simulink model "control_simulator"  (R2024b)
settings: Solver=FixedStepDiscrete  StartTime=0.0  StopTime=45  FixedStep=0.01  RelTol=1e-3
values from neighbouring files (symbols this model uses):
  Kd_dote = 0    [controller_params.m]
  Kd_dotp = 0    [controller_params.m]
  Kd_dott = 0.2    [controller_params.m]
  Kd_e = 0    [controller_params.m]
  Kd_p = 1    [controller_params.m]
  Kd_t = 0.16    [controller_params.m]
  Ki_dote = 10    [controller_params.m]
  Ki_dotp = 1.2    [controller_params.m]
  Ki_dott = 0.05    [controller_params.m]
  Ki_e = 0    [controller_params.m]
  Ki_p = 0    [controller_params.m]
  Ki_t = 0.0    (= 0)    [controller_params.m]
  Kp_dote = 5    [controller_params.m]
  Kp_dotp = 3.8    [controller_params.m]
  Kp_dott = 0.3    [controller_params.m]
  Kp_e = 1.5    [controller_params.m]
  Kp_p = 1.5    [controller_params.m]
  Kp_t = 0.4    [controller_params.m]
  max_dote = 4    [controller_params.m]
  max_dotp = 3    [controller_params.m]
  max_dott = deg2rad(15)    [controller_params.m]
  max_e = deg2rad(45)    [controller_params.m]
  max_p = deg2rad(45)    [controller_params.m]
  max_t = deg2rad(45)    [controller_params.m]
  min_dote = 0    [controller_params.m]
  min_dotp = -3    [controller_params.m]
  min_dott = -deg2rad(15)    [controller_params.m]
  min_e = -deg2rad(45)    [controller_params.m]
  min_p = -deg2rad(45)    [controller_params.m]
  min_t = -deg2rad(45)    [controller_params.m]
libraries: slpidlib x6
settings Model: Creator=bryankikuta  LastModifiedBy=bryankikuta

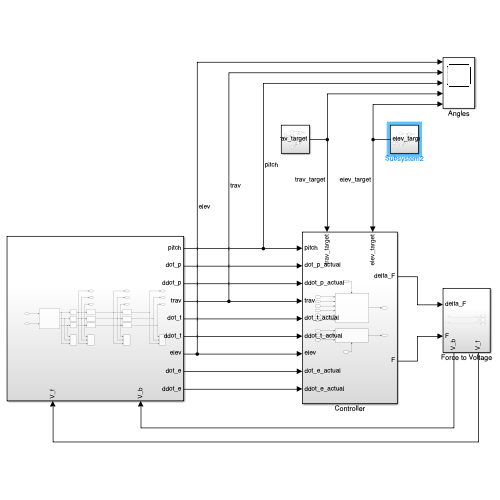
[thumbnail: Simulink's stored preview of the top-level diagram]
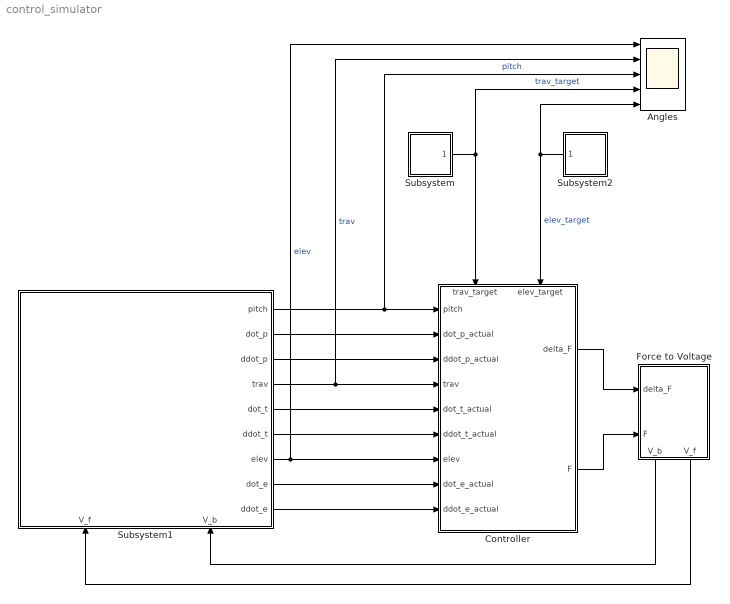
== system control_simulator ==
  Angles : Scope  NumInputPorts=5
  Controller : Subsystem
      settings: PortSchema="{\"entries\":[{\"content\":{\"sides\":[{\"content\":{\"connectorIds\":[\"In1\",\"In2\",\"In3\",\"In4\",\"In5\",\"In6\",\"In7\",\"In8\",\"In9\"]},\"type\":\"ConnectorPlacement.EquallySpacedRectSide\",\"uuid\":\"b9be8901-0178-4093-bc1f-7a19329e3ddd\"},{\"content\":{\"connectorIds\":[\"Out1\",\"Out2\"],\"side\":\"RIGHT\"},\"type\":\"ConnectorPlacement.EquallySpacedRectSide\",\"uuid\":\"79e1f72b-8678-4c9d-874f-f1aeb3aff2e8\"},{\"content\":{\"connectorIds\":[\"In10\",\"In11\"],\"side\":\"TOP\"},\"type\":\"ConnectorPlacement.EquallySpacedRectSide\",\"uuid\":\"c11cbc2b-c46d-45de-b9fa-5f1631f2c60a\"}]},\"type\":\"ConnectorPlacement.EquallySpacedConnector\",\"uuid\":\"5eabee5a-01a3-4056-9340-8a43b1588280\"}],\"packageUris\":[\"http://schema.mathworks.com/mf0/Connector/R2020b\"],\"version\":\"1.0\"}"
  Force to Voltage : Subsystem
      settings: PortSchema="{\"entries\":[{\"content\":{\"sides\":[{\"content\":{\"connectorIds\":[\"In1\",\"In2\"]},\"type\":\"ConnectorPlacement.EquallySpacedRectSide\",\"uuid\":\"6f137349-bbac-4947-af72-a88291b00c32\"},{\"content\":{\"side\":\"RIGHT\"},\"type\":\"ConnectorPlacement.EquallySpacedRectSide\",\"uuid\":\"62cbe85c-e78c-4219-9070-536950e9188e\"},{\"content\":{\"side\":\"TOP\"},\"type\":\"ConnectorPlacement.EquallySpacedRectSide\",\"uuid\":\"b2b4bc51-a272-402c-9560-9dda5e41a8e7\"},{\"content\":{\"connectorIds\":[\"Out1\",\"Out2\"],\"side\":\"BOTTOM\"},\"type\":\"ConnectorPlacement.EquallySpacedRectSide\",\"uuid\":\"97d29757-9418-4318-9369-020d2350e0e0\"}]},\"type\":\"ConnectorPlacement.EquallySpacedConnector\",\"uuid\":\"58f565a6-402e-4fc1-b947-4e751bcba226\"}],\"packageUris\":[\"http://schema.mathworks.com/mf0/Connector/R2020b\"],\"version\":\"1.0\"}"
  Subsystem : Subsystem
  Subsystem1 : Subsystem
      settings: PortSchema="{\"entries\":[{\"content\":{\"sides\":[{\"content\":{},\"type\":\"ConnectorPlacement.EquallySpacedRectSide\",\"uuid\":\"85796e1e-dc7e-47a4-94ca-9dbd2389fb42\"},{\"content\":{\"connectorIds\":[\"Out1\",\"Out2\",\"Out3\",\"Out4\",\"Out5\",\"Out6\",\"Out7\",\"Out8\",\"Out9\"],\"side\":\"RIGHT\"},\"type\":\"ConnectorPlacement.EquallySpacedRectSide\",\"uuid\":\"0966b95d-a260-4754-9670-31181c58c2b3\"},{\"content\":{\"side\":\"TOP\"},\"type\":\"ConnectorPlacement.EquallySpacedRectSide\",\"uuid\":\"e674cd1b-7e3a-4241-b627-b9ea271cb489\"},{\"content\":{\"connectorIds\":[\"In1\",\"In2\"],\"side\":\"BOTTOM\"},\"type\":\"ConnectorPlacement.EquallySpacedRectSide\",\"uuid\":\"4a7c60fe-460d-4522-942d-cbc66a60857c\"}]},\"type\":\"ConnectorPlacement.EquallySpacedConnector\",\"uuid\":\"488257c1-7be2-46d6-bbfb-c75cce3631e5\"}],\"packageUris\":[\"http://schema.mathworks.com/mf0/Connector/R2020b\"],\"version\":\"1.0\"}"
  Subsystem2 : Subsystem
      settings: PortSchema="{\"entries\":[{\"content\":{\"sides\":[{\"content\":{\"connectorIds\":[\"Out1\"]},\"type\":\"ConnectorPlacement.EquallySpacedRectSide\",\"uuid\":\"f16ebcfb-7c7e-48d0-898d-d7ef16663e42\"},{\"content\":{\"side\":\"RIGHT\"},\"type\":\"ConnectorPlacement.EquallySpacedRectSide\",\"uuid\":\"e9aec1bf-af4d-4e60-94a2-adac9fbe53b1\"},{\"content\":{\"side\":\"TOP\"},\"type\":\"ConnectorPlacement.EquallySpacedRectSide\",\"uuid\":\"bae62bc1-b0f5-4305-8efd-ec446c0d0572\"}]},\"type\":\"ConnectorPlacement.EquallySpacedConnector\",\"uuid\":\"f37ab34b-dfa4-4a7d-8642-621e1edbbf7a\"}],\"packageUris\":[\"http://schema.mathworks.com/mf0/Connector/R2020b\"],\"version\":\"1.0\"}"
  wires:
  Subsystem1/1(pitch) -> Angles/3, Controller/1(pitch)  "pitch"
  Subsystem1/4(trav) -> Angles/2, Controller/4(trav)  "trav"
  Subsystem1/7(elev) -> Angles/1, Controller/7(elev)  "elev"
  Force to Voltage/2(V_f) -> Subsystem1/1(V_f)
  Force to Voltage/1(V_b) -> Subsystem1/2(V_b)
  Subsystem1/2(dot_p) -> Controller/2(dot_p_actual)
  Subsystem1/3(ddot_p) -> Controller/3(ddot_p_actual)
  Subsystem1/5(dot_t) -> Controller/5(dot_t_actual)
  Subsystem1/6(ddot_t) -> Controller/6(ddot_t_actual)
  Subsystem1/8(dot_e) -> Controller/8(dot_e_actual)
  Subsystem1/9(ddot_e) -> Controller/9(ddot_e_actual)
  Controller/1(delta_F) -> Force to Voltage/1(delta_F)
  Controller/2(F) -> Force to Voltage/2(F)
  Subsystem/1(trav_target) -> Angles/4, Controller/10(trav_target)  "trav_target"
  Subsystem2/1(elev_target) -> Controller/11(elev_target), Angles/5  "elev_target"

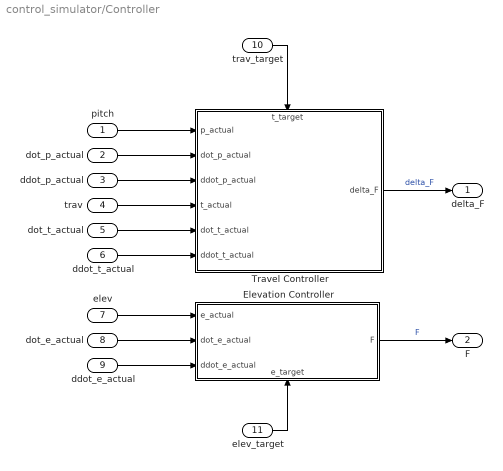
== system control_simulator/Controller ==
  pitch : Inport
  dot_p_actual : Inport  Port=2
  ddot_p_actual : Inport  Port=3
  trav : Inport  Port=4
  dot_t_actual : Inport  Port=5
  ddot_t_actual : Inport  Port=6
  elev : Inport  Port=7
  dot_e_actual : Inport  Port=8
  ddot_e_actual : Inport  Port=9
  trav_target : Inport  Port=10
  elev_target : Inport  Port=11
  Elevation Controller : Subsystem
      settings: PortSchema="{\"entries\":[{\"content\":{\"sides\":[{\"content\":{\"connectorIds\":[\"In1\",\"In2\",\"In3\"]},\"type\":\"ConnectorPlacement.EquallySpacedRectSide\",\"uuid\":\"9da0c654-dd8f-4eac-9c62-49b15265654d\"},{\"content\":{\"connectorIds\":[\"Out1\"],\"side\":\"RIGHT\"},\"type\":\"ConnectorPlacement.EquallySpacedRectSide\",\"uuid\":\"bed5ee04-0f93-4f10-b230-05550981109f\"},{\"content\":{\"side\":\"TOP\"},\"type\":\"ConnectorPlacement.EquallySpacedRectSide\",\"uuid\":\"56ea07fe-d553-41da-8d63-69b8e963b388\"},{\"content\":{\"connectorIds\":[\"In4\"],\"side\":\"BOTTOM\"},\"type\":\"ConnectorPlacement.EquallySpacedRectSide\",\"uuid\":\"e6670811-fda1-486d-a98e-2b76a62b4f3e\"}]},\"type\":\"ConnectorPlacement.EquallySpacedConnector\",\"uuid\":\"b3b4161d-49db-4a00-a039-f772733d1a23\"}],\"packageUris\":[\"http://schema.mathworks.com/mf0/Connector/R2020b\"],\"version\":\"1.0\"}"
  Travel Controller : Subsystem
      settings: PortSchema="{\"entries\":[{\"content\":{\"sides\":[{\"content\":{\"connectorIds\":[\"In1\",\"In2\",\"In3\",\"In4\",\"In5\",\"In6\"]},\"type\":\"ConnectorPlacement.EquallySpacedRectSide\",\"uuid\":\"73e9ec17-e7a6-4f85-a13a-6f8910987c35\"},{\"content\":{\"connectorIds\":[\"Out1\"],\"side\":\"RIGHT\"},\"type\":\"ConnectorPlacement.EquallySpacedRectSide\",\"uuid\":\"c5195cd8-79c4-4218-a9bb-56ca77b55f6e\"},{\"content\":{\"connectorIds\":[\"In7\"],\"side\":\"TOP\"},\"type\":\"ConnectorPlacement.EquallySpacedRectSide\",\"uuid\":\"2d754233-a1a1-48e7-852a-7aeefa75e1cb\"}]},\"type\":\"ConnectorPlacement.EquallySpacedConnector\",\"uuid\":\"9648f682-433b-4a20-950d-debe9f6c7fac\"}],\"packageUris\":[\"http://schema.mathworks.com/mf0/Connector/R2020b\"],\"version\":\"1.0\"}"
  delta_F : Outport
  F : Outport  Port=2
  wires:
  trav_target/1 -> Travel Controller/7(t_target)
  pitch/1 -> Travel Controller/1(p_actual)
  dot_t_actual/1 -> Travel Controller/5(dot_t_actual)
  ddot_p_actual/1 -> Travel Controller/3(ddot_p_actual)
  elev/1 -> Elevation Controller/1(e_actual)
  dot_p_actual/1 -> Travel Controller/2(dot_p_actual)
  Travel Controller/1(delta_F) -> delta_F/1  "delta_F"
  Elevation Controller/1(F) -> F/1  "F"
  dot_e_actual/1 -> Elevation Controller/2(dot_e_actual)
  trav/1 -> Travel Controller/4(t_actual)
  elev_target/1 -> Elevation Controller/4(e_target)
  ddot_t_actual/1 -> Travel Controller/6(ddot_t_actual)
  ddot_e_actual/1 -> Elevation Controller/3(ddot_e_actual)

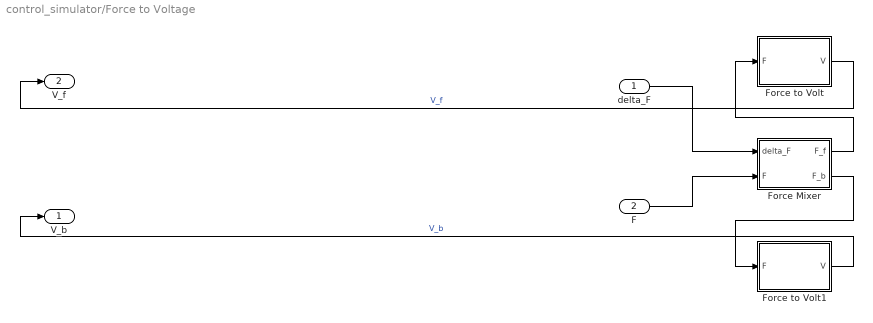
== system control_simulator/Force to Voltage ==
  delta_F : Inport
  F : Inport  Port=2
  Force Mixer : MATLAB Function  TreatAsAtomicUnit=on
  Force to Volt : MATLAB Function  TreatAsAtomicUnit=on
  Force to Volt1 : MATLAB Function  TreatAsAtomicUnit=on
  V_b : Outport
  V_f : Outport  Port=2
  wires:
  Force Mixer/2(F_b) -> Force to Volt1/1(F)
  Force to Volt1/1(V) -> V_b/1  "V_b"
  F/1 -> Force Mixer/2(F)
  delta_F/1 -> Force Mixer/1(delta_F)
  Force to Volt/1(V) -> V_f/1  "V_f"
  Force Mixer/1(F_f) -> Force to Volt/1(F)

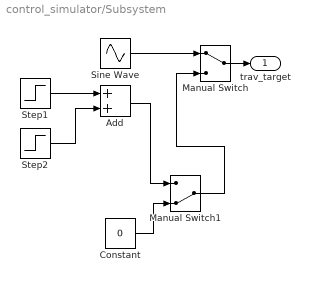
== system control_simulator/Subsystem ==
  Add : Sum
  Constant : Constant  Value=0
  Manual Switch : ManualSwitch
  Manual Switch1 : ManualSwitch  CurrentSetting=0
  Sine Wave : Sin  Amplitude=deg2rad(45)  Frequency=0.2  SampleTime=0
  Step1 : Step  Time=8  After=deg2rad(90)  SampleTime=0
  Step2 : Step  Time=25  After=deg2rad(-45)  SampleTime=0
  trav_target : Outport
  wires:
  Sine Wave/1 -> Manual Switch/1
  Manual Switch/1 -> trav_target/1
  Step1/1 -> Add/1
  Step2/1 -> Add/2
  Constant/1 -> Manual Switch1/2
  Add/1 -> Manual Switch1/1
  Manual Switch1/1 -> Manual Switch/2

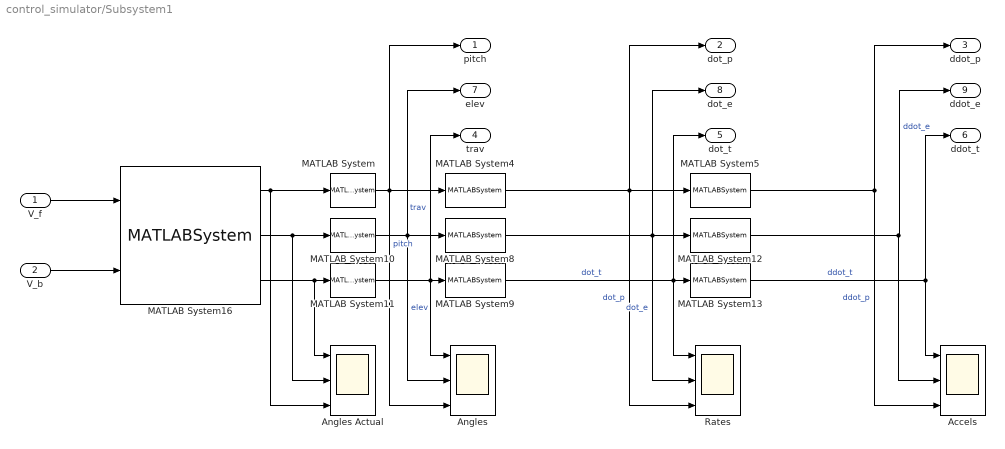
== system control_simulator/Subsystem1 ==
  V_f : Inport
  V_b : Inport  Port=2
  Accels : Scope  NumInputPorts=3
  Angles : Scope  NumInputPorts=3
  Angles Actual : Scope  NumInputPorts=3
  MATLAB System : MATLABSystem  System=MovingAverage  window_size=10  SimulateUsing=Code generation
      mask Type: MovingAverage
      mask Display:
      | disp('MovingAverage');
      | port_label('input',1,'input');
      | port_label('output',1,'avg');
  MATLAB System10 : MATLABSystem  System=MovingAverage  window_size=10  SimulateUsing=Code generation
      mask Type: MovingAverage
      mask Display:
      | disp('MovingAverage');
      | port_label('input',1,'input');
      | port_label('output',1,'avg');
  MATLAB System11 : MATLABSystem  System=MovingAverage  window_size=10  SimulateUsing=Code generation
      mask Type: MovingAverage
      mask Display:
      | disp('MovingAverage');
      | port_label('input',1,'input');
      | port_label('output',1,'avg');
  MATLAB System{4..5,8..9,12..13} (6 alike) : MATLABSystem  System=Derivative  SimulateUsing=Code generation
      mask Type: Derivative
      mask Display:
      | disp('Derivative');
      | port_label('input',1,'val');
      | port_label('output',1,'der');
  MATLAB System16 : MATLABSystem  System=HeliSystem  V_max=30  a_thrust=0.0053  b_thrust=0.0022  a_torque=0.0003  b_torque=0.0004  b_1=0.20  b_2=0.238  b_3=25.75 * 0.0254  b_4=0.0513  L_h=6.985 * 0.0254  L_a=25.75 * 0.0254  L_w=18.125 * 0.0254  g=9.81  T_stat_pitch=0.001  T_stat_elev=0.001  T_stat_trav=0.005  T_coeff_pitch=0.1  T_coeff_elev=0.1  T_coeff_trav=0.1  m_f=0.721  m_b=0.721  m_w=1.914  ax_pitch=[ -1; 0; 0 ]  ax_elev=[ 0; 1; 0 ]  ax_trav=[ 0; 0; -1 ]  F_f=[ 0; 0; -1 ]  F_b=[ 0; 0; -1 ]  T_f=[ 0; 0; 1 ]  T_b=[ 0; 0; -1 ]  pitch_init=deg2rad( 0 )  elev_init=deg2rad( -30 )  trav_init=deg2rad( 0 )  pitch_max=deg2rad( 90 )  pitch_min=deg2rad( -90 )  elev_max=deg2rad( 30 )  elev_min=deg2rad( -30 )  trav_max=deg2rad( 180 )  trav_min=deg2rad( -180 )  theta=deg2rad( 17.1 )  SimulateUsing=Code generation
      mask Type: HeliSystem
      mask Display:
      | disp('HeliSystem');
      | port_label('input',1,'V_f');
      | port_label('input',2,'V_b');
      | port_label('output',1,'pitch');
      | port_label('output',2,'elev');
      | port_label('output',3,'trav');
  Rates : Scope  NumInputPorts=3
  pitch : Outport
  dot_p : Outport  Port=2
  ddot_p : Outport  Port=3
  trav : Outport  Port=4
  dot_t : Outport  Port=5
  ddot_t : Outport  Port=6
  elev : Outport  Port=7
  dot_e : Outport  Port=8
  ddot_e : Outport  Port=9
  wires:
  V_f/1 -> MATLAB System16/1
  V_b/1 -> MATLAB System16/2
  MATLAB System10/1 -> MATLAB System8/1, Angles/2, elev/1  "elev"
  MATLAB System11/1 -> MATLAB System9/1, Angles/1, trav/1  "trav"
  MATLAB System4/1 -> Rates/3, MATLAB System5/1, dot_p/1  "dot_p"
  MATLAB System8/1 -> MATLAB System12/1, Rates/2, dot_e/1  "dot_e"
  MATLAB System9/1 -> MATLAB System13/1, Rates/1, dot_t/1  "dot_t"
  MATLAB System16/1 -> Angles Actual/3, MATLAB System/1
  MATLAB System16/2 -> Angles Actual/2, MATLAB System10/1
  MATLAB System16/3 -> Angles Actual/1, MATLAB System11/1
  MATLAB System/1 -> MATLAB System4/1, Angles/3, pitch/1  "pitch"
  MATLAB System12/1 -> Accels/2, ddot_e/1  "ddot_e"
  MATLAB System5/1 -> Accels/3, ddot_p/1  "ddot_p"
  MATLAB System13/1 -> ddot_t/1, Accels/1  "ddot_t"

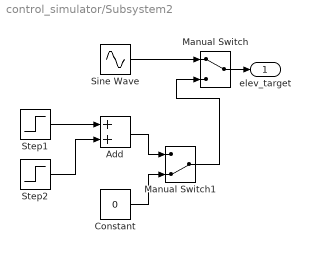
== system control_simulator/Subsystem2 ==
  Add : Sum
  Constant : Constant  Value=0
  Manual Switch : ManualSwitch
  Manual Switch1 : ManualSwitch  CurrentSetting=0
  Sine Wave : Sin  Amplitude=deg2rad(15)  Frequency=0.2  SampleTime=0
  Step1 : Step  Time=8  After=deg2rad(15)  SampleTime=0
  Step2 : Step  Time=18  After=deg2rad(-15)  SampleTime=0
  elev_target : Outport
  wires:
  Sine Wave/1 -> Manual Switch/1
  Manual Switch/1 -> elev_target/1
  Step1/1 -> Add/1
  Step2/1 -> Add/2
  Add/1 -> Manual Switch1/1
  Constant/1 -> Manual Switch1/2
  Manual Switch1/1 -> Manual Switch/2

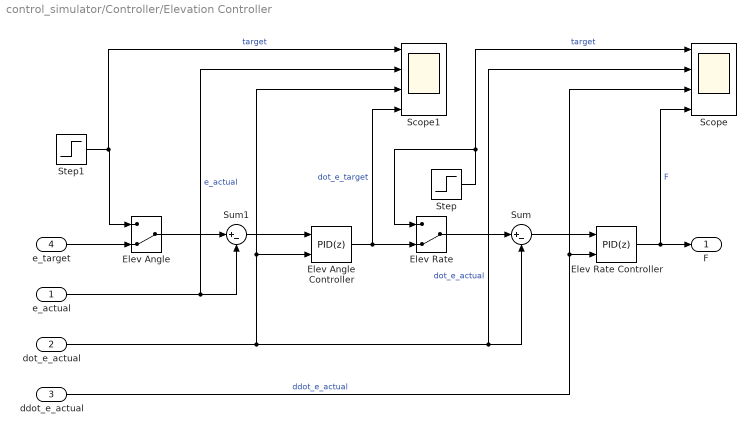
== system control_simulator/Controller/Elevation Controller ==
  e_actual : Inport
  dot_e_actual : Inport  Port=2
  ddot_e_actual : Inport  Port=3
  e_target : Inport  Port=4
  Elev Angle : ManualSwitch  CurrentSetting=0
  Elev Angle Controller : slpidlib/PID Controller  Controller=PID  Form=Parallel  TimeDomain=Discrete-time  UseExternalTs=off  SampleTime=-1  IntegratorMethod=Forward Euler  FilterMethod=Forward Euler  ControllerParametersSource=internal  P=Kp_e  I=Ki_e  UseKiTs=off  D=Kd_e  UseExternalDerivativeSource=on  N=100  UseFilter=on  TunerSelectOption=Transfer Function Based (PID Tuner App)  InitialConditionSource=internal  InitialConditionForIntegrator=0  InitialConditionForFilter=0  DifferentiatorICPrevScaledInput=0  ExternalReset=none  TrackingMode=off  Kt=1  LimitOutput=on  SatLimitsSource=internal  UpperSaturationLimit=max_e  LowerSaturationLimit=min_e  LinearizeAsGain=on  AntiWindupMode=none  Kb=1  LimitIntegrator=off  UpperIntegratorSaturationLimit=inf  LowerIntegratorSaturationLimit=-inf  POutMin=[]  POutMax=[]  IOutMin=[]  IOutMax=[]  DOutMin=[]  DOutMax=[]  NOutMin=[]  NOutMax=[]  SumOutMin=[]  SumOutMax=[]  SaturationOutMin=[]  SaturationOutMax=[]  PParamMin=[]  PParamMax=[]  IParamMin=[]  IParamMax=[]  DParamMin=[]  DParamMax=[]  NParamMin=[]  NParamMax=[]  KbParamMin=[]  KbParamMax=[]  KtParamMin=[]  KtParamMax=[]  KbOutMin=[]  KbOutMax=[]  KtOutMin=[]  KtOutMax=[]  IntegratorOutMin=[]  IntegratorOutMax=[]  FilterOutMin=[]  FilterOutMax=[]  SumI1OutMin=[]  SumI1OutMax=[]  SumI2OutMin=[]  SumI2OutMax=[]  SumI3OutMin=[]  SumI3OutMax=[]  SumI4OutMin=[]  SumI4OutMax=[]  SumDOutMin=[]  SumDOutMax=[]  DifferentiatorOutMin=[]  DifferentiatorOutMax=[]  FilterDiffOutCoefMin=[]  FilterDiffOutCoefMax=[]  ReciprocalOutMin=[]  ReciprocalOutMax=[]  SumDenOutMin=[]  SumDenOutMax=[]  SumNumOutMin=[]  SumNumOutMax=[]  DivideOutMin=[]  DivideOutMax=[]  UdiffTsProdOutMin=[]  UdiffTsProdOutMax=[]  NTsProdOutMin=[]  NTsProdOutMax=[]  UintegralTsProdOutMin=[]  UintegralTsProdOutMax=[]  UngainTsProdOutMin=[]  UngainTsProdOutMax=[]  ClampingZeroOutDataTypeStr=Inherit: Inherit via back propagation  ClampingZeroOutMin=[]  ClampingZeroOutMax=[]  FilterDenConstantOutDataTypeStr=Inherit: Inherit via back propagation  FilterDenConstantOutMin=[]  FilterDenConstantOutMax=[]  PCopyOutDataTypeStr=Inherit: Inherit via back propagation  PCopyOutMin=[]  PCopyOutMax=[]  NCopyOutDataTypeStr=Inherit: Inherit via back propagation  NCopyOutMin=[]  NCopyOutMax=[]  IntegratorContinuousStateAttributes=''  IntegratorStateMustResolveToSignalObject=off  IntegratorRTWStateStorageClass=Auto  FilterContinuousStateAttributes=''  FilterStateMustResolveToSignalObject=off  FilterRTWStateStorageClass=Auto  ParallelPVariant=InternalParameters  IdealPVariant=Disabled  IVariant=InternalParameters  DVariant=InternalParameters  IntegratorVariant=Discrete  SatVariant=Enabled  AWVariant=Passthrough  PCopyVariant=Disabled  TRVariant=Disabled  FdbkBlocksVariant=Forward  IdealPFdbkVariant=Disabled  SatFdbkVariant=Disabled  DerivativeFilterVariant=ForwardEulerFilterOnly  NVariant=InternalParameters  NCopyVariant=Disabled  FilterICVariant=InternalICsFilter  IntegratorICVariant=InternalICs  ExternalResetVariant=Disabled  TRSumVariant=Passthrough  SumFdbkVariant=Disabled  SumVariant=Sum_PID  TsampFilterVariant=InternalTs  TsampNgainVariant=Passthrough  TsampIntegralVariant=Disabled_SignalSpec  ExternalSaturationOutDataTypeStr=Inherit: Same as second input  DerivativeSourceVariant=ExternalYdot  PreIntVariant=InternalPreInt
  Elev Rate : ManualSwitch  CurrentSetting=0
  Elev Rate Controller : slpidlib/PID Controller  Controller=PID  Form=Parallel  TimeDomain=Discrete-time  UseExternalTs=off  SampleTime=-1  IntegratorMethod=Forward Euler  FilterMethod=Forward Euler  ControllerParametersSource=internal  P=Kp_dote  I=Ki_dote  UseKiTs=off  D=Kd_dote  UseExternalDerivativeSource=on  N=100  UseFilter=on  TunerSelectOption=Transfer Function Based (PID Tuner App)  InitialConditionSource=internal  InitialConditionForIntegrator=0  InitialConditionForFilter=0  DifferentiatorICPrevScaledInput=0  ExternalReset=none  TrackingMode=off  Kt=1  LimitOutput=on  SatLimitsSource=internal  UpperSaturationLimit=max_dote  LowerSaturationLimit=min_dote  LinearizeAsGain=on  AntiWindupMode=none  Kb=1  LimitIntegrator=on  UpperIntegratorSaturationLimit=max_int  LowerIntegratorSaturationLimit=min_int  POutMin=[]  POutMax=[]  IOutMin=[]  IOutMax=[]  DOutMin=[]  DOutMax=[]  NOutMin=[]  NOutMax=[]  SumOutMin=[]  SumOutMax=[]  SaturationOutMin=[]  SaturationOutMax=[]  PParamMin=[]  PParamMax=[]  IParamMin=[]  IParamMax=[]  DParamMin=[]  DParamMax=[]  NParamMin=[]  NParamMax=[]  KbParamMin=[]  KbParamMax=[]  KtParamMin=[]  KtParamMax=[]  KbOutMin=[]  KbOutMax=[]  KtOutMin=[]  KtOutMax=[]  IntegratorOutMin=[]  IntegratorOutMax=[]  FilterOutMin=[]  FilterOutMax=[]  SumI1OutMin=[]  SumI1OutMax=[]  SumI2OutMin=[]  SumI2OutMax=[]  SumI3OutMin=[]  SumI3OutMax=[]  SumI4OutMin=[]  SumI4OutMax=[]  SumDOutMin=[]  SumDOutMax=[]  DifferentiatorOutMin=[]  DifferentiatorOutMax=[]  FilterDiffOutCoefMin=[]  FilterDiffOutCoefMax=[]  ReciprocalOutMin=[]  ReciprocalOutMax=[]  SumDenOutMin=[]  SumDenOutMax=[]  SumNumOutMin=[]  SumNumOutMax=[]  DivideOutMin=[]  DivideOutMax=[]  UdiffTsProdOutMin=[]  UdiffTsProdOutMax=[]  NTsProdOutMin=[]  NTsProdOutMax=[]  UintegralTsProdOutMin=[]  UintegralTsProdOutMax=[]  UngainTsProdOutMin=[]  UngainTsProdOutMax=[]  ClampingZeroOutDataTypeStr=Inherit: Inherit via back propagation  ClampingZeroOutMin=[]  ClampingZeroOutMax=[]  FilterDenConstantOutDataTypeStr=Inherit: Inherit via back propagation  FilterDenConstantOutMin=[]  FilterDenConstantOutMax=[]  PCopyOutDataTypeStr=Inherit: Inherit via back propagation  PCopyOutMin=[]  PCopyOutMax=[]  NCopyOutDataTypeStr=Inherit: Inherit via back propagation  NCopyOutMin=[]  NCopyOutMax=[]  IntegratorContinuousStateAttributes=''  IntegratorStateMustResolveToSignalObject=off  IntegratorRTWStateStorageClass=Auto  FilterContinuousStateAttributes=''  FilterStateMustResolveToSignalObject=off  FilterRTWStateStorageClass=Auto  ParallelPVariant=InternalParameters  IdealPVariant=Disabled  IVariant=InternalParameters  DVariant=InternalParameters  IntegratorVariant=Discrete  SatVariant=Enabled  AWVariant=Passthrough  PCopyVariant=Disabled  TRVariant=Disabled  FdbkBlocksVariant=Forward  IdealPFdbkVariant=Disabled  SatFdbkVariant=Disabled  DerivativeFilterVariant=ForwardEulerFilterOnly  NVariant=InternalParameters  NCopyVariant=Disabled  FilterICVariant=InternalICsFilter  IntegratorICVariant=InternalICs  ExternalResetVariant=Disabled  TRSumVariant=Passthrough  SumFdbkVariant=Disabled  SumVariant=Sum_PID  TsampFilterVariant=InternalTs  TsampNgainVariant=Passthrough  TsampIntegralVariant=Disabled_SignalSpec  ExternalSaturationOutDataTypeStr=Inherit: Same as second input  DerivativeSourceVariant=ExternalYdot  PreIntVariant=InternalPreInt
  Scope : Scope  NumInputPorts=4
  Scope1 : Scope  NumInputPorts=4
  Step : Step  After=deg2rad(45)  SampleTime=0
  Step1 : Step  Before=deg2rad(-30)  After=deg2rad(0)  SampleTime=0
  Sum : Sum  Inputs=|+-
  Sum1 : Sum  Inputs=|+-
  F : Outport
  wires:
  Elev Rate Controller/1 -> Scope/4, F/1  "F"
  dot_e_actual/1 -> Scope1/3, Elev Angle Controller/2, Scope/2, Sum/2  "dot_e_actual"
  Sum1/1 -> Elev Angle Controller/1
  Sum/1 -> Elev Rate Controller/1
  e_actual/1 -> Scope1/2, Sum1/2  "e_actual"
  ddot_e_actual/1 -> Scope/3, Elev Rate Controller/2  "ddot_e_actual"
  Elev Angle Controller/1 -> Scope1/4, Elev Rate/2  "dot_e_target"
  Elev Rate/1 -> Sum/1
  e_target/1 -> Elev Angle/2
  Elev Angle/1 -> Sum1/1
  Step/1 -> Elev Rate/1, Scope/1  "target"
  Step1/1 -> Scope1/1, Elev Angle/1  "target"

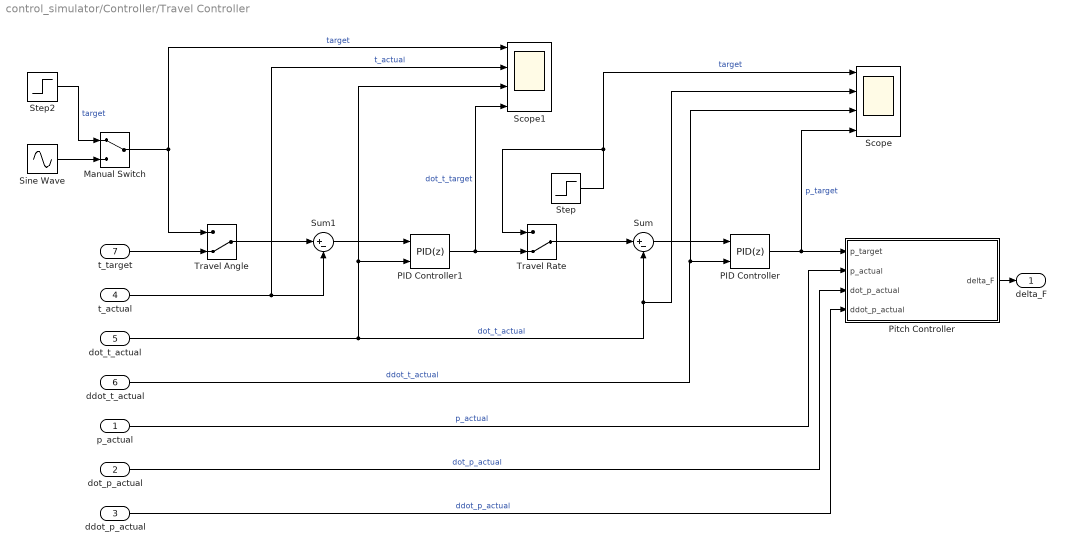
== system control_simulator/Controller/Travel Controller ==
  p_actual : Inport
  dot_p_actual : Inport  Port=2
  ddot_p_actual : Inport  Port=3
  t_actual : Inport  Port=4
  dot_t_actual : Inport  Port=5
  ddot_t_actual : Inport  Port=6
  t_target : Inport  Port=7
  Manual Switch : ManualSwitch
  PID Controller : slpidlib/PID Controller  Controller=PID  Form=Parallel  TimeDomain=Discrete-time  UseExternalTs=off  SampleTime=-1  IntegratorMethod=Forward Euler  FilterMethod=Forward Euler  ControllerParametersSource=internal  P=Kp_dott  I=Ki_dott  UseKiTs=off  D=Kd_dott  UseExternalDerivativeSource=on  N=100  UseFilter=on  TunerSelectOption=Transfer Function Based (PID Tuner App)  InitialConditionSource=internal  InitialConditionForIntegrator=0  InitialConditionForFilter=0  DifferentiatorICPrevScaledInput=0  ExternalReset=none  TrackingMode=off  Kt=1  LimitOutput=on  SatLimitsSource=internal  UpperSaturationLimit=max_dott  LowerSaturationLimit=min_dott  LinearizeAsGain=on  AntiWindupMode=none  Kb=1  LimitIntegrator=off  UpperIntegratorSaturationLimit=inf  LowerIntegratorSaturationLimit=-inf  POutMin=[]  POutMax=[]  IOutMin=[]  IOutMax=[]  DOutMin=[]  DOutMax=[]  NOutMin=[]  NOutMax=[]  SumOutMin=[]  SumOutMax=[]  SaturationOutMin=[]  SaturationOutMax=[]  PParamMin=[]  PParamMax=[]  IParamMin=[]  IParamMax=[]  DParamMin=[]  DParamMax=[]  NParamMin=[]  NParamMax=[]  KbParamMin=[]  KbParamMax=[]  KtParamMin=[]  KtParamMax=[]  KbOutMin=[]  KbOutMax=[]  KtOutMin=[]  KtOutMax=[]  IntegratorOutMin=[]  IntegratorOutMax=[]  FilterOutMin=[]  FilterOutMax=[]  SumI1OutMin=[]  SumI1OutMax=[]  SumI2OutMin=[]  SumI2OutMax=[]  SumI3OutMin=[]  SumI3OutMax=[]  SumI4OutMin=[]  SumI4OutMax=[]  SumDOutMin=[]  SumDOutMax=[]  DifferentiatorOutMin=[]  DifferentiatorOutMax=[]  FilterDiffOutCoefMin=[]  FilterDiffOutCoefMax=[]  ReciprocalOutMin=[]  ReciprocalOutMax=[]  SumDenOutMin=[]  SumDenOutMax=[]  SumNumOutMin=[]  SumNumOutMax=[]  DivideOutMin=[]  DivideOutMax=[]  UdiffTsProdOutMin=[]  UdiffTsProdOutMax=[]  NTsProdOutMin=[]  NTsProdOutMax=[]  UintegralTsProdOutMin=[]  UintegralTsProdOutMax=[]  UngainTsProdOutMin=[]  UngainTsProdOutMax=[]  ClampingZeroOutDataTypeStr=Inherit: Inherit via back propagation  ClampingZeroOutMin=[]  ClampingZeroOutMax=[]  FilterDenConstantOutDataTypeStr=Inherit: Inherit via back propagation  FilterDenConstantOutMin=[]  FilterDenConstantOutMax=[]  PCopyOutDataTypeStr=Inherit: Inherit via back propagation  PCopyOutMin=[]  PCopyOutMax=[]  NCopyOutDataTypeStr=Inherit: Inherit via back propagation  NCopyOutMin=[]  NCopyOutMax=[]  IntegratorContinuousStateAttributes=''  IntegratorStateMustResolveToSignalObject=off  IntegratorRTWStateStorageClass=Auto  FilterContinuousStateAttributes=''  FilterStateMustResolveToSignalObject=off  FilterRTWStateStorageClass=Auto  ParallelPVariant=InternalParameters  IdealPVariant=Disabled  IVariant=InternalParameters  DVariant=InternalParameters  IntegratorVariant=Discrete  SatVariant=Enabled  AWVariant=Passthrough  PCopyVariant=Disabled  TRVariant=Disabled  FdbkBlocksVariant=Forward  IdealPFdbkVariant=Disabled  SatFdbkVariant=Disabled  DerivativeFilterVariant=ForwardEulerFilterOnly  NVariant=InternalParameters  NCopyVariant=Disabled  FilterICVariant=InternalICsFilter  IntegratorICVariant=InternalICs  ExternalResetVariant=Disabled  TRSumVariant=Passthrough  SumFdbkVariant=Disabled  SumVariant=Sum_PID  TsampFilterVariant=InternalTs  TsampNgainVariant=Passthrough  TsampIntegralVariant=Disabled_SignalSpec  ExternalSaturationOutDataTypeStr=Inherit: Same as second input  DerivativeSourceVariant=ExternalYdot  PreIntVariant=InternalPreInt
  PID Controller1 : slpidlib/PID Controller  Controller=PID  Form=Parallel  TimeDomain=Discrete-time  UseExternalTs=off  SampleTime=-1  IntegratorMethod=Forward Euler  FilterMethod=Forward Euler  ControllerParametersSource=internal  P=Kp_t  I=Ki_t  UseKiTs=off  D=Kd_t  UseExternalDerivativeSource=on  N=100  UseFilter=on  TunerSelectOption=Transfer Function Based (PID Tuner App)  InitialConditionSource=internal  InitialConditionForIntegrator=0  InitialConditionForFilter=0  DifferentiatorICPrevScaledInput=0  ExternalReset=none  TrackingMode=off  Kt=1  LimitOutput=on  SatLimitsSource=internal  UpperSaturationLimit=max_t  LowerSaturationLimit=min_t  LinearizeAsGain=on  AntiWindupMode=none  Kb=1  LimitIntegrator=off  UpperIntegratorSaturationLimit=inf  LowerIntegratorSaturationLimit=-inf  POutMin=[]  POutMax=[]  IOutMin=[]  IOutMax=[]  DOutMin=[]  DOutMax=[]  NOutMin=[]  NOutMax=[]  SumOutMin=[]  SumOutMax=[]  SaturationOutMin=[]  SaturationOutMax=[]  PParamMin=[]  PParamMax=[]  IParamMin=[]  IParamMax=[]  DParamMin=[]  DParamMax=[]  NParamMin=[]  NParamMax=[]  KbParamMin=[]  KbParamMax=[]  KtParamMin=[]  KtParamMax=[]  KbOutMin=[]  KbOutMax=[]  KtOutMin=[]  KtOutMax=[]  IntegratorOutMin=[]  IntegratorOutMax=[]  FilterOutMin=[]  FilterOutMax=[]  SumI1OutMin=[]  SumI1OutMax=[]  SumI2OutMin=[]  SumI2OutMax=[]  SumI3OutMin=[]  SumI3OutMax=[]  SumI4OutMin=[]  SumI4OutMax=[]  SumDOutMin=[]  SumDOutMax=[]  DifferentiatorOutMin=[]  DifferentiatorOutMax=[]  FilterDiffOutCoefMin=[]  FilterDiffOutCoefMax=[]  ReciprocalOutMin=[]  ReciprocalOutMax=[]  SumDenOutMin=[]  SumDenOutMax=[]  SumNumOutMin=[]  SumNumOutMax=[]  DivideOutMin=[]  DivideOutMax=[]  UdiffTsProdOutMin=[]  UdiffTsProdOutMax=[]  NTsProdOutMin=[]  NTsProdOutMax=[]  UintegralTsProdOutMin=[]  UintegralTsProdOutMax=[]  UngainTsProdOutMin=[]  UngainTsProdOutMax=[]  ClampingZeroOutDataTypeStr=Inherit: Inherit via back propagation  ClampingZeroOutMin=[]  ClampingZeroOutMax=[]  FilterDenConstantOutDataTypeStr=Inherit: Inherit via back propagation  FilterDenConstantOutMin=[]  FilterDenConstantOutMax=[]  PCopyOutDataTypeStr=Inherit: Inherit via back propagation  PCopyOutMin=[]  PCopyOutMax=[]  NCopyOutDataTypeStr=Inherit: Inherit via back propagation  NCopyOutMin=[]  NCopyOutMax=[]  IntegratorContinuousStateAttributes=''  IntegratorStateMustResolveToSignalObject=off  IntegratorRTWStateStorageClass=Auto  FilterContinuousStateAttributes=''  FilterStateMustResolveToSignalObject=off  FilterRTWStateStorageClass=Auto  ParallelPVariant=InternalParameters  IdealPVariant=Disabled  IVariant=InternalParameters  DVariant=InternalParameters  IntegratorVariant=Discrete  SatVariant=Enabled  AWVariant=Passthrough  PCopyVariant=Disabled  TRVariant=Disabled  FdbkBlocksVariant=Forward  IdealPFdbkVariant=Disabled  SatFdbkVariant=Disabled  DerivativeFilterVariant=ForwardEulerFilterOnly  NVariant=InternalParameters  NCopyVariant=Disabled  FilterICVariant=InternalICsFilter  IntegratorICVariant=InternalICs  ExternalResetVariant=Disabled  TRSumVariant=Passthrough  SumFdbkVariant=Disabled  SumVariant=Sum_PID  TsampFilterVariant=InternalTs  TsampNgainVariant=Passthrough  TsampIntegralVariant=Disabled_SignalSpec  ExternalSaturationOutDataTypeStr=Inherit: Same as second input  DerivativeSourceVariant=ExternalYdot  PreIntVariant=InternalPreInt
  Pitch Controller : Subsystem
  Scope : Scope  NumInputPorts=4
  Scope1 : Scope  NumInputPorts=4
  Sine Wave : Sin  Amplitude=deg2rad(45)  Frequency=0.1  SampleTime=0
  Step : Step  After=deg2rad(45)  SampleTime=0
  Step2 : Step  After=deg2rad(45)  SampleTime=0
  Sum : Sum  Inputs=|+-
  Sum1 : Sum  Inputs=|+-
  Travel Angle : ManualSwitch  CurrentSetting=0
  Travel Rate : ManualSwitch  CurrentSetting=0
  delta_F : Outport
  wires:
  dot_t_actual/1 -> Scope1/3, PID Controller1/2, Scope/2, Sum/2  "dot_t_actual"
  p_actual/1 -> Pitch Controller/2(p_actual)  "p_actual"
  ddot_t_actual/1 -> Scope/3, PID Controller/2  "ddot_t_actual"
  PID Controller/1 -> Scope/4, Pitch Controller/1(p_target)  "p_target"
  t_actual/1 -> Scope1/2, Sum1/2  "t_actual"
  Pitch Controller/1(delta_F) -> delta_F/1
  ddot_p_actual/1 -> Pitch Controller/4(ddot_p_actual)  "ddot_p_actual"
  Sum1/1 -> PID Controller1/1
  dot_p_actual/1 -> Pitch Controller/3(dot_p_actual)  "dot_p_actual"
  Travel Angle/1 -> Sum1/1
  t_target/1 -> Travel Angle/2
  Step/1 -> Travel Rate/1, Scope/1  "target"
  Manual Switch/1 -> Travel Angle/1, Scope1/1  "target"
  Sum/1 -> PID Controller/1
  PID Controller1/1 -> Scope1/4, Travel Rate/2  "dot_t_target"
  Travel Rate/1 -> Sum/1
  Step2/1 -> Manual Switch/1  "target"
  Sine Wave/1 -> Manual Switch/2

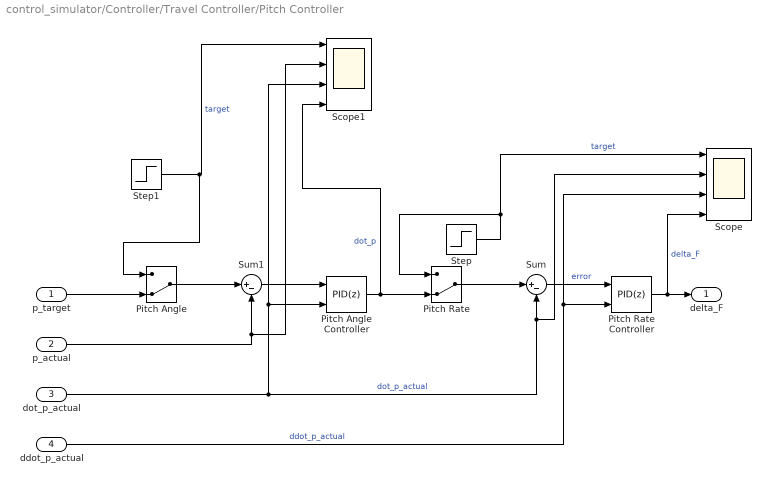
== system control_simulator/Controller/Travel Controller/Pitch Controller ==
  p_target : Inport
  p_actual : Inport  Port=2
  dot_p_actual : Inport  Port=3
  ddot_p_actual : Inport  Port=4
  Pitch Angle : ManualSwitch  CurrentSetting=0
  Pitch Angle Controller : slpidlib/PID Controller  Controller=PID  Form=Parallel  TimeDomain=Discrete-time  UseExternalTs=off  SampleTime=-1  IntegratorMethod=Forward Euler  FilterMethod=Forward Euler  ControllerParametersSource=internal  P=Kp_p  I=Ki_p  UseKiTs=off  D=Kd_p  UseExternalDerivativeSource=on  N=100  UseFilter=on  TunerSelectOption=Transfer Function Based (PID Tuner App)  InitialConditionSource=internal  InitialConditionForIntegrator=0  InitialConditionForFilter=0  DifferentiatorICPrevScaledInput=0  ExternalReset=none  TrackingMode=off  Kt=1  LimitOutput=on  SatLimitsSource=internal  UpperSaturationLimit=max_p  LowerSaturationLimit=min_p  LinearizeAsGain=on  AntiWindupMode=none  Kb=1  LimitIntegrator=off  UpperIntegratorSaturationLimit=inf  LowerIntegratorSaturationLimit=-inf  POutMin=[]  POutMax=[]  IOutMin=[]  IOutMax=[]  DOutMin=[]  DOutMax=[]  NOutMin=[]  NOutMax=[]  SumOutMin=[]  SumOutMax=[]  SaturationOutMin=[]  SaturationOutMax=[]  PParamMin=[]  PParamMax=[]  IParamMin=[]  IParamMax=[]  DParamMin=[]  DParamMax=[]  NParamMin=[]  NParamMax=[]  KbParamMin=[]  KbParamMax=[]  KtParamMin=[]  KtParamMax=[]  KbOutMin=[]  KbOutMax=[]  KtOutMin=[]  KtOutMax=[]  IntegratorOutMin=[]  IntegratorOutMax=[]  FilterOutMin=[]  FilterOutMax=[]  SumI1OutMin=[]  SumI1OutMax=[]  SumI2OutMin=[]  SumI2OutMax=[]  SumI3OutMin=[]  SumI3OutMax=[]  SumI4OutMin=[]  SumI4OutMax=[]  SumDOutMin=[]  SumDOutMax=[]  DifferentiatorOutMin=[]  DifferentiatorOutMax=[]  FilterDiffOutCoefMin=[]  FilterDiffOutCoefMax=[]  ReciprocalOutMin=[]  ReciprocalOutMax=[]  SumDenOutMin=[]  SumDenOutMax=[]  SumNumOutMin=[]  SumNumOutMax=[]  DivideOutMin=[]  DivideOutMax=[]  UdiffTsProdOutMin=[]  UdiffTsProdOutMax=[]  NTsProdOutMin=[]  NTsProdOutMax=[]  UintegralTsProdOutMin=[]  UintegralTsProdOutMax=[]  UngainTsProdOutMin=[]  UngainTsProdOutMax=[]  ClampingZeroOutDataTypeStr=Inherit: Inherit via back propagation  ClampingZeroOutMin=[]  ClampingZeroOutMax=[]  FilterDenConstantOutDataTypeStr=Inherit: Inherit via back propagation  FilterDenConstantOutMin=[]  FilterDenConstantOutMax=[]  PCopyOutDataTypeStr=Inherit: Inherit via back propagation  PCopyOutMin=[]  PCopyOutMax=[]  NCopyOutDataTypeStr=Inherit: Inherit via back propagation  NCopyOutMin=[]  NCopyOutMax=[]  IntegratorContinuousStateAttributes=''  IntegratorStateMustResolveToSignalObject=off  IntegratorRTWStateStorageClass=Auto  FilterContinuousStateAttributes=''  FilterStateMustResolveToSignalObject=off  FilterRTWStateStorageClass=Auto  ParallelPVariant=InternalParameters  IdealPVariant=Disabled  IVariant=InternalParameters  DVariant=InternalParameters  IntegratorVariant=Discrete  SatVariant=Enabled  AWVariant=Passthrough  PCopyVariant=Disabled  TRVariant=Disabled  FdbkBlocksVariant=Forward  IdealPFdbkVariant=Disabled  SatFdbkVariant=Disabled  DerivativeFilterVariant=ForwardEulerFilterOnly  NVariant=InternalParameters  NCopyVariant=Disabled  FilterICVariant=InternalICsFilter  IntegratorICVariant=InternalICs  ExternalResetVariant=Disabled  TRSumVariant=Passthrough  SumFdbkVariant=Disabled  SumVariant=Sum_PID  TsampFilterVariant=InternalTs  TsampNgainVariant=Passthrough  TsampIntegralVariant=Disabled_SignalSpec  ExternalSaturationOutDataTypeStr=Inherit: Same as second input  DerivativeSourceVariant=ExternalYdot  PreIntVariant=InternalPreInt
  Pitch Rate : ManualSwitch  CurrentSetting=0
  Pitch Rate Controller : slpidlib/PID Controller  Controller=PID  Form=Parallel  TimeDomain=Discrete-time  UseExternalTs=off  SampleTime=-1  IntegratorMethod=Forward Euler  FilterMethod=Forward Euler  ControllerParametersSource=internal  P=Kp_dotp  I=Ki_dotp  UseKiTs=off  D=Kd_dotp  UseExternalDerivativeSource=on  N=100  UseFilter=on  TunerSelectOption=Transfer Function Based (PID Tuner App)  InitialConditionSource=internal  InitialConditionForIntegrator=0  InitialConditionForFilter=0  DifferentiatorICPrevScaledInput=0  ExternalReset=none  TrackingMode=off  Kt=1  LimitOutput=on  SatLimitsSource=internal  UpperSaturationLimit=max_dotp  LowerSaturationLimit=min_dotp  LinearizeAsGain=on  AntiWindupMode=none  Kb=1  LimitIntegrator=off  UpperIntegratorSaturationLimit=inf  LowerIntegratorSaturationLimit=-inf  POutMin=[]  POutMax=[]  IOutMin=[]  IOutMax=[]  DOutMin=[]  DOutMax=[]  NOutMin=[]  NOutMax=[]  SumOutMin=[]  SumOutMax=[]  SaturationOutMin=[]  SaturationOutMax=[]  PParamMin=[]  PParamMax=[]  IParamMin=[]  IParamMax=[]  DParamMin=[]  DParamMax=[]  NParamMin=[]  NParamMax=[]  KbParamMin=[]  KbParamMax=[]  KtParamMin=[]  KtParamMax=[]  KbOutMin=[]  KbOutMax=[]  KtOutMin=[]  KtOutMax=[]  IntegratorOutMin=[]  IntegratorOutMax=[]  FilterOutMin=[]  FilterOutMax=[]  SumI1OutMin=[]  SumI1OutMax=[]  SumI2OutMin=[]  SumI2OutMax=[]  SumI3OutMin=[]  SumI3OutMax=[]  SumI4OutMin=[]  SumI4OutMax=[]  SumDOutMin=[]  SumDOutMax=[]  DifferentiatorOutMin=[]  DifferentiatorOutMax=[]  FilterDiffOutCoefMin=[]  FilterDiffOutCoefMax=[]  ReciprocalOutMin=[]  ReciprocalOutMax=[]  SumDenOutMin=[]  SumDenOutMax=[]  SumNumOutMin=[]  SumNumOutMax=[]  DivideOutMin=[]  DivideOutMax=[]  UdiffTsProdOutMin=[]  UdiffTsProdOutMax=[]  NTsProdOutMin=[]  NTsProdOutMax=[]  UintegralTsProdOutMin=[]  UintegralTsProdOutMax=[]  UngainTsProdOutMin=[]  UngainTsProdOutMax=[]  ClampingZeroOutDataTypeStr=Inherit: Inherit via back propagation  ClampingZeroOutMin=[]  ClampingZeroOutMax=[]  FilterDenConstantOutDataTypeStr=Inherit: Inherit via back propagation  FilterDenConstantOutMin=[]  FilterDenConstantOutMax=[]  PCopyOutDataTypeStr=Inherit: Inherit via back propagation  PCopyOutMin=[]  PCopyOutMax=[]  NCopyOutDataTypeStr=Inherit: Inherit via back propagation  NCopyOutMin=[]  NCopyOutMax=[]  IntegratorContinuousStateAttributes=''  IntegratorStateMustResolveToSignalObject=off  IntegratorRTWStateStorageClass=Auto  FilterContinuousStateAttributes=''  FilterStateMustResolveToSignalObject=off  FilterRTWStateStorageClass=Auto  ParallelPVariant=InternalParameters  IdealPVariant=Disabled  IVariant=InternalParameters  DVariant=InternalParameters  IntegratorVariant=Discrete  SatVariant=Enabled  AWVariant=Passthrough  PCopyVariant=Disabled  TRVariant=Disabled  FdbkBlocksVariant=Forward  IdealPFdbkVariant=Disabled  SatFdbkVariant=Disabled  DerivativeFilterVariant=ForwardEulerFilterOnly  NVariant=InternalParameters  NCopyVariant=Disabled  FilterICVariant=InternalICsFilter  IntegratorICVariant=InternalICs  ExternalResetVariant=Disabled  TRSumVariant=Passthrough  SumFdbkVariant=Disabled  SumVariant=Sum_PID  TsampFilterVariant=InternalTs  TsampNgainVariant=Passthrough  TsampIntegralVariant=Disabled_SignalSpec  ExternalSaturationOutDataTypeStr=Inherit: Same as second input  DerivativeSourceVariant=ExternalYdot  PreIntVariant=InternalPreInt
  Scope : Scope  NumInputPorts=4
  Scope1 : Scope  NumInputPorts=4
  Step : Step  After=deg2rad(45)  SampleTime=0
  Step1 : Step  After=deg2rad(30)  SampleTime=0
  Sum : Sum  Inputs=|+-
  Sum1 : Sum  Inputs=|+-
  delta_F : Outport
  wires:
  Pitch Rate Controller/1 -> Scope/4, delta_F/1  "delta_F"
  dot_p_actual/1 -> Scope1/3, Pitch Angle Controller/2, Scope/2, Sum/2  "dot_p_actual"
  Sum/1 -> Pitch Rate Controller/1  "error"
  p_actual/1 -> Scope1/2, Sum1/2
  ddot_p_actual/1 -> Scope/3, Pitch Rate Controller/2  "ddot_p_actual"
  Pitch Angle Controller/1 -> Scope1/4, Pitch Rate/2  "dot_p"
  Pitch Rate/1 -> Sum/1
  Sum1/1 -> Pitch Angle Controller/1
  Step/1 -> Pitch Rate/1, Scope/1  "target"
  Step1/1 -> Pitch Angle/1, Scope1/1  "target"
  p_target/1 -> Pitch Angle/2
  Pitch Angle/1 -> Sum1/1

== matlab function control_simulator/Force to Voltage/Force Mixer ==
  data: delta_F input; F input; F_f output; F_b output
function [F_f, F_b] = fcn(delta_F, F)
    F_f = (F + delta_F) / 2;
    F_b = (F - delta_F) / 2;
end

== matlab function control_simulator/Force to Voltage/Force to Volt1 ==
  data: F input; V output
function V = fcn(F)
    a = 0.0053;
    b = 0.0022;
    c = -abs(F);

    V = (-b + sqrt(b^2 - 4*a*c)) / (2*a);

    if F < 0
        V = -V;
    end
end

== matlab function control_simulator/Force to Voltage/Force to Volt ==
  data: F input; V output
function V = fcn(F)
    a = 0.0053;
    b = 0.0022;
    c = -abs(F);

    V = (-b + sqrt(b^2 - 4*a*c)) / (2*a);

    if F < 0
        V = -V;
    end
end
